simulink model "spid_antiwindup"  (R2020b)
settings: Solver=VariableStepAuto  StartTime=0.0  StopTime=150  RelTol=1e-3
values from neighbouring files (symbols this model uses):
  kp_cc_strejc = (1.35 / alpha_cc_strejc )*(1 + ((0.18 * tau_cc_strejc)/ (1 - tau_cc_strejc)))    [lab1.m]    (also in lab4.m)
  td_cc_strejc = ((0.37 - 0.37* tau_cc_strejc)/(1 - 0.81 * tau_cc_strejc)) * l_cc_strejc    [lab1.m]    (also in lab4.m)
  ti_cc_strejc = ((2.50 - 2.0 * tau_cc_strejc)/(1 - 0.39 * tau_cc_strejc)) * l_cc_strejc    [lab1.m]    (also in lab4.m)
undefined symbols (not defined in the file or in its folder): plant_1
settings Model: Creator=rafael  LastModifiedBy=rafael

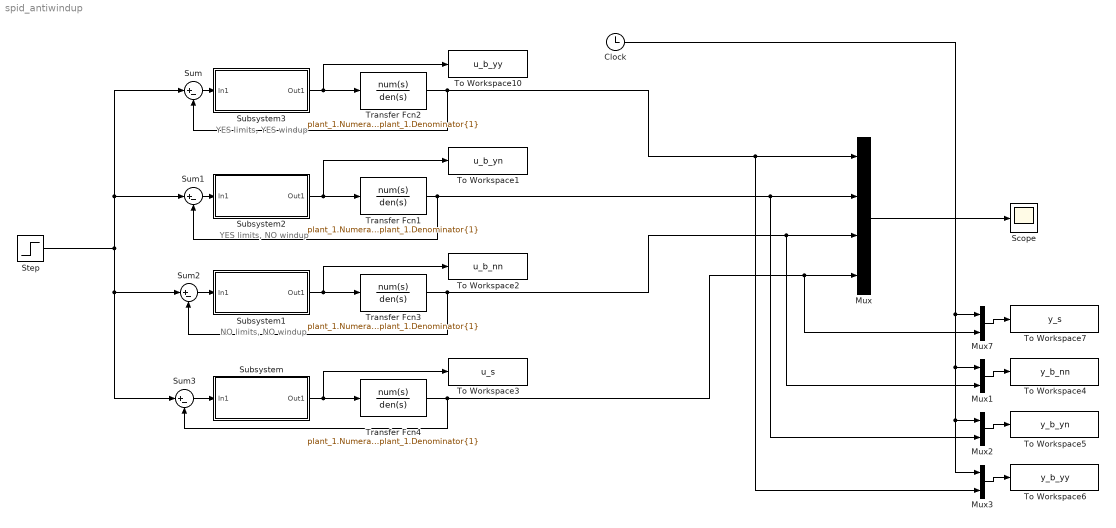
== system spid_antiwindup ==
  note: NO limits, NO windup
  note: YES limits, NO windup
  note: YES limits, YES windup
  Clock : Clock
  Mux : Mux
  Mux{1..3,7} (4 alike) : Mux  Inputs=2
  Scope : Scope
  Step : Step  SampleTime=0
  Subsystem : Subsystem  mask{kp=kp_cc_strejc, ti=ti_cc_strejc, td=td_cc_strejc}
      mask prompts: kp "Proportional gain (kp)"; ti "Integral time (ti)"; td "Derrivative_time (td)"
      mask help: u(s)=kp*(1 + (1/ti)/s + td*s)
      mask Help: /*No help for now*/
      mask Display: disp(' standardPID '), port_label('input',1,'e'), port_label('output',1,'u')
  Subsystem1 : Subsystem  mask{kp=kp_cc_strejc, ti=ti_cc_strejc, td=td_cc_strejc, t_t=1000000, s_lim=1000}
      mask prompts: kp "Proportional gain (kp)"; ti "Integral time (ti)"; td "Derrivative_time (td)"; t_t "T_f for the anti windup"; s_lim "Saturation_limit"
      mask help:
      | u(s)=kp*(1 + (1/ti)/s + td*s)
      | with anti windup and saturation
      mask Help: /*No help for now*/
      mask Display: disp(' standardPID\n better '), port_label('input',1,'e'), port_label('output',1,'u')
  Subsystem2 : Subsystem  mask{kp=kp_cc_strejc, ti=ti_cc_strejc, td=td_cc_strejc, t_t=100000, s_lim=0.8}
      mask prompts: kp "Proportional gain (kp)"; ti "Integral time (ti)"; td "Derrivative_time (td)"; t_t "T_f for the anti windup"; s_lim "Saturation_limit"
      mask help:
      | u(s)=kp*(1 + (1/ti)/s + td*s)
      | with anti windup and saturation
      mask Help: /*No help for now*/
      mask Display: disp(' standardPID\n better '), port_label('input',1,'e'), port_label('output',1,'u')
  Subsystem3 : Subsystem  mask{kp=kp_cc_strejc, ti=ti_cc_strejc, td=td_cc_strejc, t_t=sqrt(ti_cc_strejc*td_cc_strejc), s_lim=0.8}
      mask prompts: kp "Proportional gain (kp)"; ti "Integral time (ti)"; td "Derrivative_time (td)"; t_t "T_f for the anti windup"; s_lim "Saturation_limit"
      mask help:
      | u(s)=kp*(1 + (1/ti)/s + td*s)
      | with anti windup and saturation
      mask Help: /*No help for now*/
      mask Display: disp(' standardPID\n better '), port_label('input',1,'e'), port_label('output',1,'u')
  Sum{,1..3} (4 alike) : Sum  Inputs=|+-
  To Workspace1 : ToWorkspace  VariableName=u_b_yn  SampleTime=-1
      settings: Save2DSignal=2-D array (concatenate along first dimension)
  To Workspace10 : ToWorkspace  VariableName=u_b_yy  SampleTime=-1
      settings: Save2DSignal=2-D array (concatenate along first dimension)
  To Workspace2 : ToWorkspace  VariableName=u_b_nn  SampleTime=-1
      settings: Save2DSignal=2-D array (concatenate along first dimension)
  To Workspace3 : ToWorkspace  VariableName=u_s  SampleTime=-1
      settings: Save2DSignal=2-D array (concatenate along first dimension)
  To Workspace4 : ToWorkspace  VariableName=y_b_nn  SampleTime=-1
      settings: Save2DSignal=2-D array (concatenate along first dimension)
  To Workspace5 : ToWorkspace  VariableName=y_b_yn  SampleTime=-1
      settings: Save2DSignal=2-D array (concatenate along first dimension)
  To Workspace6 : ToWorkspace  VariableName=y_b_yy  SampleTime=-1
      settings: Save2DSignal=2-D array (concatenate along first dimension)
  To Workspace7 : ToWorkspace  VariableName=y_s  SampleTime=-1
      settings: Save2DSignal=2-D array (concatenate along first dimension)
  Transfer Fcn{1..4} (4 alike) : TransferFcn  Numerator=plant_1.Numerator{1}  Denominator=plant_1.Denominator{1}
  wires:
  Subsystem3/1(Out1) -> Transfer Fcn2/1, To Workspace10/1
  Subsystem2/1(Out1) -> Transfer Fcn1/1, To Workspace1/1
  Subsystem1/1(Out1) -> Transfer Fcn3/1, To Workspace2/1
  Subsystem/1(Out1) -> Transfer Fcn4/1, To Workspace3/1
  Transfer Fcn4/1 -> Mux7/2, Mux/4, Sum3/2
  Mux7/1 -> To Workspace7/1
  Mux1/1 -> To Workspace4/1
  Transfer Fcn3/1 -> Mux/3, Mux1/2, Sum2/2
  Mux/1 -> Scope/1
  Transfer Fcn1/1 -> Mux/2, Mux2/2, Sum1/2
  Mux2/1 -> To Workspace5/1
  Clock/1 -> Mux3/1, Mux2/1, Mux1/1, Mux7/1
  Mux3/1 -> To Workspace6/1
  Transfer Fcn2/1 -> Mux/1, Mux3/2, Sum/2
  Sum3/1 -> Subsystem/1(In1)
  Sum2/1 -> Subsystem1/1(In1)
  Sum1/1 -> Subsystem2/1(In1)
  Sum/1 -> Subsystem3/1(In1)
  Step/1 -> Sum3/1, Sum2/1, Sum1/1, Sum/1

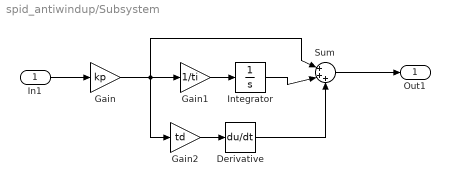
== system spid_antiwindup/Subsystem ==
  In1 : Inport
  Derivative : Derivative
  Gain : Gain  Gain=kp
  Gain1 : Gain  Gain=1/ti
  Gain2 : Gain  Gain=td
  Integrator : Integrator
  Sum : Sum  Inputs=|+++
  Out1 : Outport
  wires:
  Sum/1 -> Out1/1
  In1/1 -> Gain/1
  Derivative/1 -> Sum/3
  Gain/1 -> Gain2/1, Gain1/1, Sum/1
  Gain2/1 -> Derivative/1
  Integrator/1 -> Sum/2
  Gain1/1 -> Integrator/1

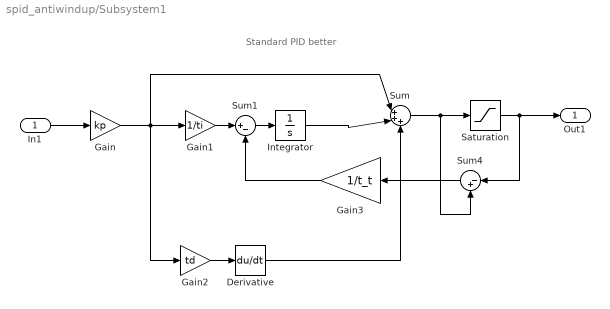
== system spid_antiwindup/Subsystem1 ==
  note: Standard PID better
  In1 : Inport
  Derivative : Derivative
  Gain : Gain  Gain=kp
  Gain1 : Gain  Gain=1/ti
  Gain2 : Gain  Gain=td
  Gain3 : Gain  Gain=1/t_t
  Integrator : Integrator
  Saturation : Saturate  UpperLimit=s_lim  LowerLimit=-s_lim
  Sum : Sum  Inputs=|+++
  Sum1 : Sum  Inputs=|+-
  Sum4 : Sum  Inputs=|-+
  Out1 : Outport
  wires:
  In1/1 -> Gain/1
  Derivative/1 -> Sum/3
  Gain/1 -> Gain2/1, Gain1/1, Sum/1
  Gain2/1 -> Derivative/1
  Integrator/1 -> Sum/2
  Sum4/1 -> Gain3/1
  Sum/1 -> Sum4/2, Saturation/1
  Saturation/1 -> Sum4/1, Out1/1
  Gain3/1 -> Sum1/2
  Gain1/1 -> Sum1/1
  Sum1/1 -> Integrator/1

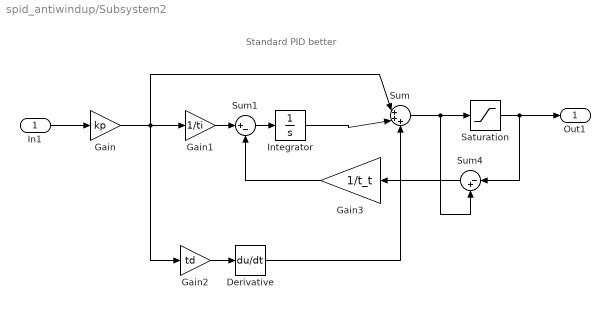
== system spid_antiwindup/Subsystem2 ==
  note: Standard PID better
  In1 : Inport
  Derivative : Derivative
  Gain : Gain  Gain=kp
  Gain1 : Gain  Gain=1/ti
  Gain2 : Gain  Gain=td
  Gain3 : Gain  Gain=1/t_t
  Integrator : Integrator
  Saturation : Saturate  UpperLimit=s_lim  LowerLimit=-s_lim
  Sum : Sum  Inputs=|+++
  Sum1 : Sum  Inputs=|+-
  Sum4 : Sum  Inputs=|-+
  Out1 : Outport
  wires:
  In1/1 -> Gain/1
  Derivative/1 -> Sum/3
  Gain/1 -> Gain2/1, Gain1/1, Sum/1
  Gain2/1 -> Derivative/1
  Integrator/1 -> Sum/2
  Sum4/1 -> Gain3/1
  Sum/1 -> Sum4/2, Saturation/1
  Saturation/1 -> Sum4/1, Out1/1
  Gain3/1 -> Sum1/2
  Gain1/1 -> Sum1/1
  Sum1/1 -> Integrator/1

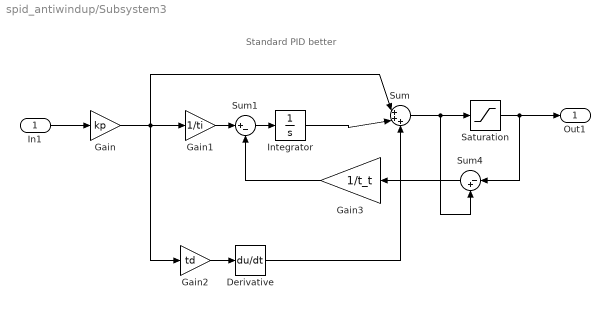
== system spid_antiwindup/Subsystem3 ==
  note: Standard PID better
  In1 : Inport
  Derivative : Derivative
  Gain : Gain  Gain=kp
  Gain1 : Gain  Gain=1/ti
  Gain2 : Gain  Gain=td
  Gain3 : Gain  Gain=1/t_t
  Integrator : Integrator
  Saturation : Saturate  UpperLimit=s_lim  LowerLimit=-s_lim
  Sum : Sum  Inputs=|+++
  Sum1 : Sum  Inputs=|+-
  Sum4 : Sum  Inputs=|-+
  Out1 : Outport
  wires:
  In1/1 -> Gain/1
  Derivative/1 -> Sum/3
  Gain/1 -> Gain2/1, Gain1/1, Sum/1
  Gain2/1 -> Derivative/1
  Integrator/1 -> Sum/2
  Sum4/1 -> Gain3/1
  Sum/1 -> Sum4/2, Saturation/1
  Saturation/1 -> Sum4/1, Out1/1
  Gain3/1 -> Sum1/2
  Gain1/1 -> Sum1/1
  Sum1/1 -> Integrator/1
